simulink model "simulink2masses"  (R2015a)
settings: Solver=ode15s  StartTime=0.0  StopTime=y_final  RelTol=1e-3
values from neighbouring files (symbols this model uses):
  c1 = str2num(get(handles.c1t,'String'))    [guiproject.m]
  k1 = str2num(get(handles.k1t,'String'))    [guiproject.m]
  k2 = str2num(get(handles.k2t,'String'))    [guiproject.m]
  m1 = str2num(get(handles.m1t,'String'))    [guiproject.m]
  m2 = str2num(get(handles.m2t,'String'))    [guiproject.m]
  y_final = str2num(get(handles.y_finalt,'String'))    [guiproject.m]
settings Model: Creator=b00058261  LastModifiedBy=b00058261

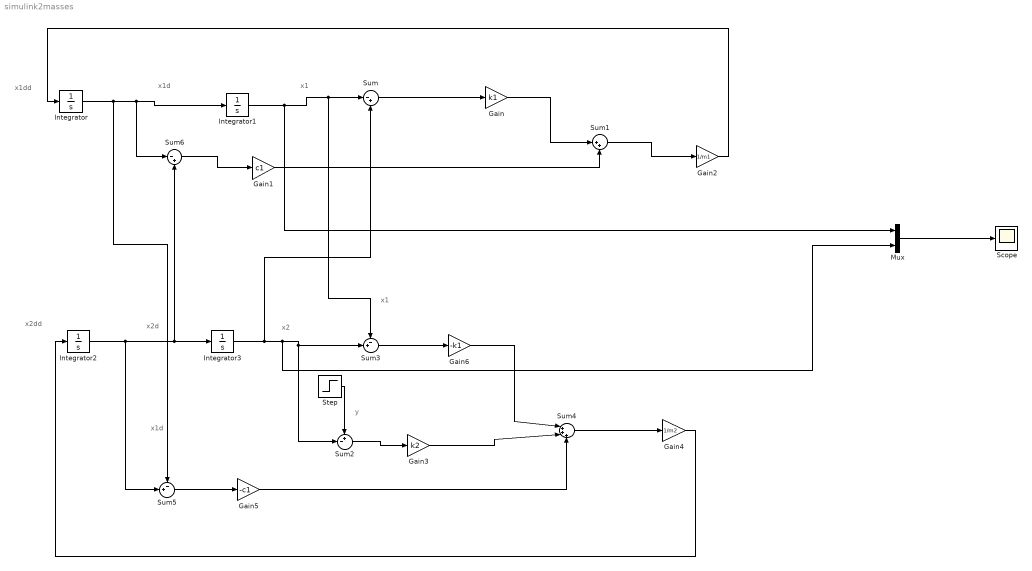
== system simulink2masses ==
  note: x1
  note: x1d
  note: x1dd
  note: y
  note: x1d
  note: x1
  note: x2
  note: x2d
  note: x2dd
  Gain : Gain  Gain=k1
  Gain1 : Gain  Gain=c1
  Gain2 : Gain  Gain=1/m1
  Gain3 : Gain  Gain=k2
  Gain4 : Gain  Gain=1/m2
  Gain5 : Gain  Gain=-c1
  Gain6 : Gain  Gain=-k1
  Integrator{,1..3} (4 alike) : Integrator
  Mux : Mux  Inputs=2
  Scope : Scope
      settings: SaveName=mass_2
  Step : Step  Time=0  After=y_final  SampleTime=0
  Sum : Sum  Inputs=|-+
  Sum1 : Sum  Inputs=|++
  Sum2 : Sum  Inputs=+-|
  Sum3 : Sum  Inputs=-+|
  Sum4 : Sum  Inputs=|+++
  Sum5 : Sum  Inputs=-+|
  Sum6 : Sum  Inputs=|-+
  wires:
  Integrator2/1 -> Sum6/2, Integrator3/1, Sum5/2
  Sum5/1 -> Gain5/1
  Integrator3/1 -> Sum/2, Mux/2, Sum2/2, Sum3/2
  Sum3/1 -> Gain6/1
  Sum2/1 -> Gain3/1
  Gain6/1 -> Sum4/1
  Gain3/1 -> Sum4/2
  Gain5/1 -> Sum4/3
  Sum4/1 -> Gain4/1
  Gain4/1 -> Integrator2/1
  Integrator/1 -> Sum5/1, Sum6/1, Integrator1/1
  Sum6/1 -> Gain1/1
  Integrator1/1 -> Mux/1, Sum3/1, Sum/1
  Sum/1 -> Gain/1
  Gain/1 -> Sum1/1
  Gain1/1 -> Sum1/2
  Sum1/1 -> Gain2/1
  Gain2/1 -> Integrator/1
  Step/1 -> Sum2/1
  Mux/1 -> Scope/1
